simulink model "LCK_0112"  (R2018b)
settings: Solver=FixedStepDiscrete  StartTime=0.0  StopTime=inf  FixedStep=0.01  RelTol=1e-3
PostLoadFcn:
  | if any(exist('dsrtsu_mdlpostloadfcn', 'file') ~= 0), dsrtsu_mdlpostloadfcn('Execute', bdroot); end
values from neighbouring files (symbols this model uses):
  C_DEG2RAD = 0.0175    [LCK_Macro.sldd]
  C_KPH2MPS = 0.2778    [LCK_Macro.sldd]
  C_NEARZERO = 0.0001    [LCK_Macro.sldd]
  C_ONE = 1.0    [LCK_Macro.sldd]
  C_RAD2DEG = 57.2958    [LCK_Macro.sldd]
  C_ZERO = 0.0    [LCK_Macro.sldd]
  k_accel_pedal_pos_per_speed_x : value not decoded    [LCK_LogicPara.sldd]
  k_accel_pedal_pos_per_speed_z : value not decoded    [LCK_LogicPara.sldd]
  k_brake_suprress_hold = 1000.0    [LCK_LogicPara.sldd]
  k_driver_appl_torque_filt = 50.0    [LCK_LogicPara.sldd]
  k_driver_suppression_hold_time = 3000.0    [LCK_LogicPara.sldd]
  k_hands_on_wheel_hold_msec = 500.0    [LCK_LogicPara.sldd]
  k_hands_on_wheel_torque_hi = 0.2    [LCK_LogicPara.sldd]
  k_hands_on_wheel_torque_lo = 0.15    [LCK_LogicPara.sldd]
  k_handsoff_delay_cycles = 50.0    [LCK_LogicPara.sldd]
  k_handsoff_torq_Lo_CR = 0.3    [LCK_LogicPara.sldd]
  k_handson_delay_cycles = 5.0    [LCK_LogicPara.sldd]
  k_HighAccel_suppress_hold = 3000.0    [LCK_LogicPara.sldd]
  k_HLR_suprress_hold = 3000.0    [LCK_LogicPara.sldd]
  k_hs_StrAng_CR_threshold_z : value not decoded    [LCK_LogicPara.sldd]
  k_LC_Exit_Switch = 0.0    [LCK_LogicPara.sldd]
  k_LCG_Configured = 1.0    [LCK_LogicPara.sldd]
  k_LCK_A0_Rdy2Act_UseConst = 0.0    [LCK_LogicPara.sldd]
  k_LCK_A0Fac_ActSta : value not decoded    [LCK_CtrlPara.sldd]
  k_LCK_A0Fac_DrvStm : value not decoded    [LCK_CtrlPara.sldd]
  k_LCK_A0Shift_LftCurv : value not decoded    [LCK_CtrlPara.sldd]
  k_LCK_A0Shift_RgtCurv : value not decoded    [LCK_CtrlPara.sldd]
  k_LCK_A0Shift_StraLan = 0.0    [LCK_CtrlPara.sldd]
  k_LCK_A0ShiftFac_Dy_LftCurv : value not decoded    [LCK_CtrlPara.sldd]
  k_LCK_A0ShiftFac_Dy_RgtCurv : value not decoded    [LCK_CtrlPara.sldd]
  k_LCK_A0ShiftFac_Vspd : value not decoded    [LCK_CtrlPara.sldd]
  k_LCK_accel_inhibit_thold = 35.0    [LCK_LogicPara.sldd]
  k_LCK_Active2Ready_Mask = 255.0    [LCK_LogicPara.sldd]
  k_LCK_CvatRateBks : value not decoded    [LCK_CtrlPara.sldd]
  k_LCK_CvatrBks : value not decoded    [LCK_CtrlPara.sldd]
  k_LCK_DFac_Dy : value not decoded    [LCK_CtrlPara.sldd]
  k_LCK_DFac_Dy_Curv : value not decoded    [LCK_CtrlPara.sldd]
  k_LCK_DFac_HaCurCen : value not decoded    [LCK_CtrlPara.sldd]
  k_LCK_DFac_HaCurSid : value not decoded    [LCK_CtrlPara.sldd]
  k_LCK_DFac_HadCurCen : value not decoded    [LCK_CtrlPara.sldd]
  k_LCK_DFac_HadCurSid : value not decoded    [LCK_CtrlPara.sldd]
  k_LCK_DFac_HadStrCen : value not decoded    [LCK_CtrlPara.sldd]
  k_LCK_DFac_HadStrSid : value not decoded    [LCK_CtrlPara.sldd]
  k_LCK_DFac_HaStrCen : value not decoded    [LCK_CtrlPara.sldd]
  k_LCK_DFac_HaStrSid : value not decoded    [LCK_CtrlPara.sldd]
  k_LCK_DFac_Rad : value not decoded    [LCK_CtrlPara.sldd]
  k_LCK_DFac_SA_CurCen : value not decoded    [LCK_CtrlPara.sldd]
  k_LCK_DFac_SA_CurSid : value not decoded    [LCK_CtrlPara.sldd]
  k_LCK_DFac_SA_StrCen : value not decoded    [LCK_CtrlPara.sldd]
  k_LCK_DFac_SA_StrSid : value not decoded    [LCK_CtrlPara.sldd]
  k_LCK_DFac_SS_CurCen : value not decoded    [LCK_CtrlPara.sldd]
  k_LCK_DFac_SS_CurSid : value not decoded    [LCK_CtrlPara.sldd]
  k_LCK_DFac_SS_StrCen : value not decoded    [LCK_CtrlPara.sldd]
  k_LCK_DFac_SS_StrSid : value not decoded    [LCK_CtrlPara.sldd]
  k_LCK_DFac_Vspd : value not decoded    [LCK_CtrlPara.sldd]
  k_LCK_DlyTm_DrvStim = 0.2    [LCK_CtrlPara.sldd]
  k_LCK_DTermMax = 2.0    [LCK_CtrlPara.sldd]
  k_LCK_DyBks_Curv : value not decoded    [LCK_CtrlPara.sldd]
  k_LCK_Enable_POOnly = 1.0    [LCK_LogicPara.sldd]
  k_LCK_Entry_DistBuffer = 0.1    [LCK_LogicPara.sldd]
  k_LCK_Fac_Vspd2RngThr_FalRec = 0.23    [LCK_CtrlPara.sldd]
  k_LCK_Ffw_CvatSwh = 0.0    [LCK_CtrlPara.sldd]
  k_LCK_Ffw_DyBks : value not decoded    [LCK_CtrlPara.sldd]
  k_LCK_Ffw_TimCon_CmdFlt = 0.0    [LCK_CtrlPara.sldd]
  k_LCK_FfwDeltaFac_Rad_Lft : value not decoded    [LCK_CtrlPara.sldd]
  k_LCK_FfwDeltaFac_Rad_Rgt : value not decoded    [LCK_CtrlPara.sldd]
  k_LCK_FfwDeltaFac_Vspd : value not decoded    [LCK_CtrlPara.sldd]
  k_LCK_FfwFac_CvatRate_Lft : value not decoded    [LCK_CtrlPara.sldd]
  k_LCK_FfwFac_CvatRate_Rgt : value not decoded    [LCK_CtrlPara.sldd]
  k_LCK_FfwFac_Dy : value not decoded    [LCK_CtrlPara.sldd]
  k_LCK_FfwFac_Rad_Lft : value not decoded    [LCK_CtrlPara.sldd]
  k_LCK_FfwFac_Rad_Rgt : value not decoded    [LCK_CtrlPara.sldd]
  k_LCK_FfwFac_Vspd : value not decoded    [LCK_CtrlPara.sldd]
  k_LCK_FfwTorq_Cvat : value not decoded    [LCK_CtrlPara.sldd]
  k_LCK_HAFac_ActSta : value not decoded    [LCK_CtrlPara.sldd]
  k_LCK_HAFac_DrvStm : value not decoded    [LCK_CtrlPara.sldd]
  k_LCK_HaloTime = 2000.0    [LCK_LogicPara.sldd]
  k_LCK_HaloTime_Switch = 0.0    [LCK_LogicPara.sldd]
  k_LCK_HARFac_ActSta : value not decoded    [LCK_CtrlPara.sldd]
  k_LCK_HARFac_DrvStm : value not decoded    [LCK_CtrlPara.sldd]
  k_LCK_Hed_DyBks : value not decoded    [LCK_CtrlPara.sldd]
  k_LCK_HedAngDiffX : value not decoded    [LCK_CtrlPara.sldd]
  k_LCK_HedAngRateDiffX : value not decoded    [LCK_CtrlPara.sldd]
  k_LCK_HndsOnWhel_DlyTm_Idl2Rdy = 0.0    [LCK_LogicPara.sldd]
  k_LCK_host_veh_width = 1.86    [LCK_LogicPara.sldd]
  k_LCK_Idle2Ready_Mask = 239.0    [LCK_LogicPara.sldd]
  k_LCK_Junc_SusTime = 1.0    [LCK_LogicPara.sldd]
  k_LCK_KpKdDecSlopeLmt = 10.0    [LCK_CtrlPara.sldd]
  k_LCK_KpKdIncSlopeLmt = 5.0    [LCK_CtrlPara.sldd]
  k_LCK_Lat_Ctrl_DFac_Lft = 1.0    [LCK_CtrlPara.sldd]
  k_LCK_Lat_Ctrl_DFac_Rgt = 1.05    [LCK_CtrlPara.sldd]
  k_LCK_Lat_Ctrl_Kd = 0.8    [LCK_CtrlPara.sldd]
  k_LCK_Lat_Ctrl_Ki = 0.5    [LCK_CtrlPara.sldd]
  k_LCK_Lat_Ctrl_Kp = 0.7    [LCK_CtrlPara.sldd]
  k_LCK_Lat_Ctrl_Kp_NearGain = 0.7    [LCK_CtrlPara.sldd]
  k_LCK_Lat_Ctrl_PFac_Lft = 1.0    [LCK_CtrlPara.sldd]
  k_LCK_Lat_Ctrl_PFac_Rgt = 1.05    [LCK_CtrlPara.sldd]
  k_LCK_Lat_Ctrl_TimCon_CmdFlt = 5.0    [LCK_CtrlPara.sldd]
  k_LCK_Lat_DFac_Rad : value not decoded    [LCK_CtrlPara.sldd]
  k_LCK_Lat_DFac_SS_Cur : value not decoded    [LCK_CtrlPara.sldd]
  k_LCK_Lat_DFac_SS_Str : value not decoded    [LCK_CtrlPara.sldd]
  k_LCK_Lat_DFac_Vspd : value not decoded    [LCK_CtrlPara.sldd]
  k_LCK_Lat_DyBks : value not decoded    [LCK_CtrlPara.sldd]
  k_LCK_Lat_IFac_Rad : value not decoded    [LCK_CtrlPara.sldd]
  k_LCK_Lat_IFac_Vspd : value not decoded    [LCK_CtrlPara.sldd]
  k_LCK_Lat_ILmtFac_Dy_CurvLan : value not decoded    [LCK_CtrlPara.sldd]
  k_LCK_Lat_ILmtFac_Dy_StraLan : value not decoded    [LCK_CtrlPara.sldd]
  k_LCK_Lat_ILmtFac_Rad : value not decoded    [LCK_CtrlPara.sldd]
  k_LCK_Lat_ILmtFac_Rad_NearGain = 1.0    [LCK_CtrlPara.sldd]
  k_LCK_Lat_ILmtFac_Vspd_CurvLan : value not decoded    [LCK_CtrlPara.sldd]
  k_LCK_Lat_ILmtFac_Vspd_StraLan : value not decoded    [LCK_CtrlPara.sldd]
  k_LCK_Lat_ITermLmt_Dy = 1.0    [LCK_CtrlPara.sldd]
  k_LCK_Lat_KpKdDecSlopeLmt = 10.0    [LCK_CtrlPara.sldd]
  k_LCK_Lat_KpKdIncSlopeLmt = 10.0    [LCK_CtrlPara.sldd]
  k_LCK_Lat_PFac_Dy_InnLftCur : value not decoded    [LCK_CtrlPara.sldd]
  k_LCK_Lat_PFac_Dy_InnRgtCur : value not decoded    [LCK_CtrlPara.sldd]
  k_LCK_Lat_PFac_Dy_OutLftCur : value not decoded    [LCK_CtrlPara.sldd]
  k_LCK_Lat_PFac_Dy_OutRgtCur : value not decoded    [LCK_CtrlPara.sldd]
  k_LCK_Lat_PFac_Dy_Str : value not decoded    [LCK_CtrlPara.sldd]
  k_LCK_Lat_PFac_Rad : value not decoded    [LCK_CtrlPara.sldd]
  ... (+153 more)
undefined symbols (not defined in the file or in its folder): k_LCK_CurvBks, K_LCK_SPA0A1A2_LMRngCmp_y
libraries: LateralControl_fcns_lib x58, simulink x24
(part 8 of 45)

== system LCK_0112/Lateral_Control_Module/Adas_Lateral_Control_LCK_Core/Module 4 ==
  SPP_A0 : Inport
  SPP_A1 : Inport  Port=2
  SPP_A2 : Inport  Port=3
  SPP_A3 : Inport  Port=4
  Actual_Hed_Ang_Rate : Inport  Port=5
  Sig_Wekng_Factor : Inport  Port=6
  Road_Radius : Inport  Port=7
  Str_Flag : Inport  Description=_GWMH9P3.LCK.000_669_  Port=8
  Cur_Flag : Inport  Description=_GWMH9P3.LCK.000_669_  Port=9
  Vspd : Inport  Port=10
  Add : Sum
  Bus Selector4 : BusSelector  OutputSignals=A0_Wekng_Fac,HA_Wekng_Fac,HAR_Wekng_Fac
  C_KPH2MPS : Gain  Description=_GWMAB30P2.LCK.000_1299_  Gain=C_KPH2MPS
  C_RAD2DEG : Gain  Gain=C_RAD2DEG
  Constant2 : Constant  Description=_GWMAB30P3.LCK.000_155_  OutDataTypeStr=single
  Lookup_Table : Lookup_n-D  NumberOfTableDimensions=1  BreakpointsForDimension1=k_LCK_RadBks  Table=[0.4 0.4 0.5 0.5 0.5 0.6 0.6 0.6 0.7 0.7 0.7 0.8 0.8 1.2]  ExtrapMethod=Clip  InternalRulePriority=Speed  RndMeth=Simplest  InputSameDT=on
  Product : Product
  Product1 : Product
  Product10 : Product  Description=_GWMAB30P2.LCK.000_1355_  RndMeth=Zero
  Product2 : Product
  Product3 : Product  Description=_GWMAB30P2.LCK.000_1346_  RndMeth=Zero
  Product4 : Product  Description=_GWMAB30P2.LCK.000_1352_  RndMeth=Zero
  Product5 : Product  Description=_GWMAB30P2.LCK.000_1353_  Inputs=4  RndMeth=Zero
  Product6 : Product  Description=_GWMAB30P2.LCK.000_1354_  Inputs=3  RndMeth=Zero
  Product7 : Product  Description=_GWMAB30P2.LCK.000_1346_  Inputs=3  RndMeth=Zero
  Sum1 : Sum  Description=_GWMAB30P2.LCK.000_1363_  Inputs=++++
  Switch{,1..2,4} (4 alike) : Switch  Description=_GWMAB30P2.LCK.000_1368_  Threshold=0.5
  Trigonometric Function : Trigonometry  Description=_GWMAB30P2.LCK.000_1369_  Operator=atan
  Trigonometric Function1 : Trigonometry  Description=_GWMAB30P2.LCK.000_1370_
  k_LCK_A0ShiftFac_Dy_LftCurv : Lookup_n-D  NumberOfTableDimensions=1  BreakpointsForDimension1=k_LCK_DyBks_Curv  BreakpointsForDimension2=K_LCK_SPA0A1A2_LMRngCmp_y  Table=k_LCK_A0ShiftFac_Dy_LftCurv  ExtrapMethod=Clip  InternalRulePriority=Speed  RndMeth=Simplest  InputSameDT=on
  k_LCK_A0ShiftFac_Dy_RgtCurv : Lookup_n-D  NumberOfTableDimensions=1  BreakpointsForDimension1=k_LCK_DyBks_Curv  BreakpointsForDimension2=K_LCK_SPA0A1A2_LMRngCmp_y  Table=k_LCK_A0ShiftFac_Dy_RgtCurv  ExtrapMethod=Clip  InternalRulePriority=Speed  RndMeth=Simplest  InputSameDT=on
  k_LCK_A0ShiftFac_Vspd : Lookup_n-D  NumberOfTableDimensions=1  BreakpointsForDimension1=k_LCK_VspdBks  BreakpointsForDimension2=K_LCK_SPA0A1A2_LMRngCmp_y  Table=k_LCK_A0ShiftFac_Vspd  ExtrapMethod=Clip  InternalRulePriority=Speed  RndMeth=Simplest  InputSameDT=on
  k_LCK_A0Shift_LftCurv : Lookup_n-D  NumberOfTableDimensions=1  BreakpointsForDimension1=k_LCK_RadBks  BreakpointsForDimension2=K_LCK_SPA0A1A2_LMRngCmp_y  Table=k_LCK_A0Shift_LftCurv  ExtrapMethod=Clip  InternalRulePriority=Speed  RndMeth=Simplest  InputSameDT=on
  k_LCK_A0Shift_RgtCurv : Lookup_n-D  NumberOfTableDimensions=1  BreakpointsForDimension1=k_LCK_RadBks  BreakpointsForDimension2=K_LCK_SPA0A1A2_LMRngCmp_y  Table=k_LCK_A0Shift_RgtCurv  ExtrapMethod=Clip  InternalRulePriority=Speed  RndMeth=Simplest  InputSameDT=on
  k_LCK_A0Shift_StraLan : Constant  Description=_GWMAB30P3.LCK.000_155_  Value=k_LCK_A0Shift_StraLan
  Dy_1 : Outport  Description=_GWMH9P3.LCK.000_786_
  Dy_0 : Outport  Description=_GWMH9P3.LCK.000_786_  Port=2
  Lat_Rate : Outport  Description=_GWMH9P3.LCK.000_786_  Port=3
  Hed_Ang : Outport  Description=_GWMH9P3.LCK.000_786_  Port=4
  Hed_Ang_Rat : Outport  Description=_GWMH9P3.LCK.000_786_  Port=5
  wires:
  Bus Selector4/2 -> Product1/2  "<HA_Wekng_Fac>"
  Bus Selector4/3 -> Product2/1  "<HAR_Wekng_Fac>"
  Actual_Hed_Ang_Rate/1 -> Product2/2
  Product2/1 -> Hed_Ang_Rat/1
  Trigonometric Function1/1 -> Product10/2
  Trigonometric Function/1 -> C_RAD2DEG/1, Trigonometric Function1/1
  Product1/1 -> Trigonometric Function/1
  C_KPH2MPS/1 -> Product10/1, Product3/1
  Product4/1 -> Sum1/2
  Product3/1 -> Product5/4, Product5/2, Product5/3, Product6/2, Product6/3, Product4/2
  SPP_A2/1 -> Product6/1
  SPP_A1/1 -> Product4/1, Product1/1
  SPP_A3/1 -> Product5/1
  Product5/1 -> Sum1/4
  Product6/1 -> Sum1/3
  Lookup_Table/1 -> Product3/2
  Sig_Wekng_Factor/1 -> Bus Selector4/1
  Bus Selector4/1 -> Product/2  "<A0_Wekng_Fac>"
  Sum1/1 -> Dy_1/1
  Product7/1 -> Add/2
  Vspd/1 -> C_KPH2MPS/1, k_LCK_A0ShiftFac_Vspd/1
  Product/1 -> Dy_0/1, Sum1/1
  Road_Radius/1 -> [Road_Radius], k_LCK_A0Shift_LftCurv/1, k_LCK_A0Shift_RgtCurv/1
  k_LCK_A0Shift_StraLan/1 -> Switch/1
  Str_Flag/1 -> Switch/2, [Straight_Lane_Flag]
  k_LCK_A0Shift_LftCurv/1 -> Switch1/1
  k_LCK_A0Shift_RgtCurv/1 -> Switch1/3
  Switch1/1 -> Switch/3
  [Straight_Lane_Flag] -> Switch2/2
  Constant2/1 -> Switch2/1
  Cur_Flag/1 -> Switch4/2, [Left_Curve_Lane_Flag]
  SPP_A0/1 -> Add/1, k_LCK_A0ShiftFac_Dy_RgtCurv/1, k_LCK_A0ShiftFac_Dy_LftCurv/1
  Switch4/1 -> Switch2/3
  Switch2/1 -> Product7/1
  Switch/1 -> Product7/2
  k_LCK_A0ShiftFac_Vspd/1 -> Product7/3
  Add/1 -> Product/1
  [Road_Radius] -> Lookup_Table/1
  [Left_Curve_Lane_Flag] -> Switch1/2
  k_LCK_A0ShiftFac_Dy_RgtCurv/1 -> Switch4/3
  k_LCK_A0ShiftFac_Dy_LftCurv/1 -> Switch4/1
  Product10/1 -> Lat_Rate/1
  C_RAD2DEG/1 -> Hed_Ang/1

== system LCK_0112/Lateral_Control_Module/Adas_Lateral_Control_LCK_Core/Module 5 ==
  Vspd : Inport
  SP_A2 : Inport  Port=2
  SP_A3 : Inport  Port=3
  Abs : Abs  Description=_GWMAB30P2.LCK.000_1340_
  Abs1 : Abs  Description=_GWMAB30P2.LCK.000_1340_
  Abs3 : Abs
  C_KPH2MPS : Gain  Description=_GWMAB30P2.LCK.000_1299_  Gain=C_KPH2MPS
  C_NEARZERO : Constant  Description=_GWMAB30P3.LCK.000_154_  Value=C_NEARZERO
  Compare To Constant : simulink/Logic and Bit Operations/Compare To Constant  Description=_GWMAB30P4.LCK.000_309_  relop=<  const=0.00004  OutDataTypeStr=uint8
  Compare To Constant1 : simulink/Logic and Bit Operations/Compare To Constant  Description=_GWMAB30P4.LCK.000_309_  relop=<  const=0.00004  OutDataTypeStr=uint8
  Constant1 : Constant  Description=_GWMAB30P3.LCK.000_155_  Value=0  OutDataTypeStr=single
  Constant2 : Constant  Description=_GWMAB30P3.LCK.000_155_  OutDataTypeStr=single
  Constant22 : Constant  Description=_GWMAB30P3.LCK.000_155_  Value=0  OutDataTypeStr=single
  Divide : Product  Description=_GWMAB30P3.LCK.000_157_  Inputs=*/
  First_Order_Lag_Filter_LIB : LateralControl_fcns_lib/First_Order_Lag_Filter_LIB  SystemSampleTime=-1
  Gain : Gain  Description=_GWMAB30P2.LCK.000_1342_  Gain=2
  Gain2 : Gain  Description=_GWMAB30P2.LCK.000_1343_  Gain=6
  Gain3 : Gain  Description=_GWMAB30P2.LCK.000_1343_  Gain=6
  Lookup_Table : Lookup_n-D  NumberOfTableDimensions=1  BreakpointsForDimension1=k_LCK_RadBks  Table=[0.4 0.4 0.5 0.5 0.5 0.6 0.6 0.6 0.7 0.7 0.7 0.8 0.8 1.2]  ExtrapMethod=Clip  InternalRulePriority=Speed  RndMeth=Simplest  InputSameDT=on
  ML_TIME_MSEC : Constant  Description=_GWMAB30P3.LCK.000_166_  Value=ML_TIME_MSEC
  MinMax2 : MinMax  Description=_GWMAB30P3.LCK.000_167_  Function=max  Inputs=2
  Product1 : Product  Description=_GWMAB30P2.LCK.000_1347_  RndMeth=Zero
  Product3 : Product  Description=_GWMAB30P2.LCK.000_1346_  RndMeth=Zero
  Sum : Sum  Description=_GWMAB30P2.LCK.000_1362_
  Switch : Switch  Description=_GWMAB30P2.LCK.000_1368_  Threshold=0.5
  Switch1 : Switch  Description=_GWMAB30P2.LCK.000_1368_  Threshold=0.5
  Terminator2 : Terminator
  Terminator3 : Terminator
  k_LCK_TimCon_RadFlt : Constant  Description=_GWMAB30P3.LCK.000_168_  Value=k_LCK_TimCon_RadFlt
  Road_Radius : Outport
  Curvature_0 : Outport  Port=2
  Curvature_1 : Outport  Port=3
  Curvature_Rate : Outport  Port=4
  wires:
  First_Order_Lag_Filter_LIB/1 -> Lookup_Table/1, Road_Radius/1
  SP_A2/1 -> Gain/1
  Constant22/1 -> Switch/1
  Compare To Constant/1 -> Switch/2
  Abs/1 -> Compare To Constant/1
  Divide/1 -> First_Order_Lag_Filter_LIB/1, Terminator3/1  "Road_Radius"
  Constant2/1 -> Divide/1
  MinMax2/1 -> Divide/2
  C_NEARZERO/1 -> MinMax2/2
  ML_TIME_MSEC/1 -> First_Order_Lag_Filter_LIB/3
  k_LCK_TimCon_RadFlt/1 -> First_Order_Lag_Filter_LIB/2
  Abs3/1 -> MinMax2/1
  Switch/1 -> Abs3/1
  Sum/1 -> Abs1/1, Switch1/3
  Constant1/1 -> Switch1/1
  Compare To Constant1/1 -> Switch1/2
  Abs1/1 -> Compare To Constant1/1
  SP_A3/1 -> Gain3/1, Gain2/1
  Gain/1 -> Switch/3, Sum/1, Curvature_0/1, Abs/1
  Gain2/1 -> Curvature_Rate/1, Product1/1
  Product3/1 -> Product1/2
  Product1/1 -> Sum/2
  Switch1/1 -> Curvature_1/1
  Lookup_Table/1 -> Product3/2
  C_KPH2MPS/1 -> Product3/1
  Vspd/1 -> C_KPH2MPS/1
  Gain3/1 -> Terminator2/1  "Curvature_Rate"
